simulink model "PendulumSim"  (Simulink 7.7)
settings: Solver=ode5  StartTime=0.0  StopTime=550  FixedStep=.01  RelTol=1e-3
values from neighbouring files (symbols this model uses):
  B = 2*Zeta*natFreq*J    [PendulumDamping.m]
  g = 9.81    [PendulumDamping.m]
  J = m*g*rBar/natFreq^2    [PendulumDamping.m]
  m = 0.0820142    [PendulumDamping.m]
  rBar = 0.0857    [PendulumDamping.m]
undefined symbols (not defined in the file or in its folder): Tf_alpha
settings Model: Creator=pturpel  LastModifiedBy=pturpel

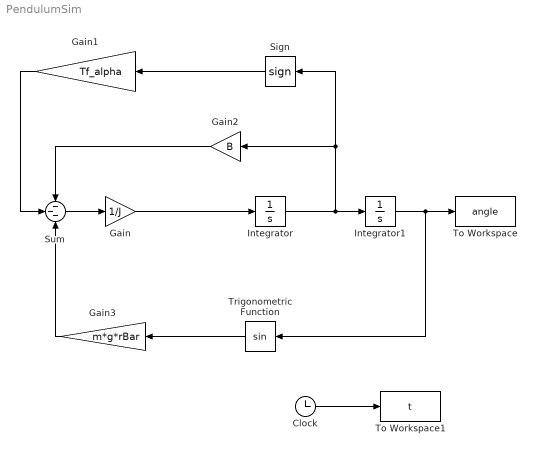
== system PendulumSim ==
  Clock : Clock
      settings: Decimation=10
  Gain : Gain  Gain=1/J
  Gain1 : Gain  Gain=Tf_alpha
  Gain2 : Gain  Gain=B
  Gain3 : Gain  Gain=m*g*rBar
  Integrator : Integrator
  Integrator1 : Integrator  InitialCondition=.8535
  Sign : Signum
  Sum : Sum  Inputs=---
  To Workspace : ToWorkspace  VariableName=angle  SampleTime=-1  SaveFormat=Array
  To Workspace1 : ToWorkspace  VariableName=t  SampleTime=-1  SaveFormat=Array
  Trigonometric Function : Trigonometry
  wires:
  Integrator/1 -> Integrator1/1, Sign/1, Gain2/1
  Sign/1 -> Gain1/1
  Sum/1 -> Gain/1
  Gain/1 -> Integrator/1
  Gain2/1 -> Sum/1
  Integrator1/1 -> To Workspace/1, Trigonometric Function/1
  Gain3/1 -> Sum/3
  Clock/1 -> To Workspace1/1
  Gain1/1 -> Sum/2
  Trigonometric Function/1 -> Gain3/1
